simulink model "DHM"  (R2022a)
settings: Solver=FixedStepDiscrete  StartTime=0.0  StopTime=10.0  FixedStep=0.01  RelTol=1e-3
libraries: simulink x8, DoorHndDriver x4, DoorHndReq x4, DoorHndPosSts x4
(part 2 of 2)

== stateflow chart DHM/DHM_Step_sys/DHM/DoorHndSetSts ==
  state DrvDoorHndSet [parallel]
    settings: executionOrder=1
    (default) -> (junction 2)
    DrvDoorHndSet -> (junction 2)
    (junction 2) -> (junction 3) [order 1] : [hasChanged(SI_e_DrvDoorHndSet)]
    (junction 2) -> (junction 4) [order 2]
    (junction 3) -> (junction 39) : {SL_e_DrvDoorHndSetBackup = ...
        | SI_e_DrvDoorHndSet;}
    (junction 4) -> (junction 5) [order 1] : [SL_e_DrvDoorHndSetBackup == 4]
    (junction 4) -> (junction 43) [order 2]
    (junction 5) -> (junction 27)
    (junction 43) -> (junction 17) [order 1] : [SL_e_DrvDoorHndSetBackup == 3]
    (junction 27) -> (junction 6) [order 1] : [SI_m_FLDoorHndPosSts == Hnd_Unfold]
    (junction 43) -> (junction 26) [order 2]
    (junction 17) -> (junction 14) : {SO_b_DrvDoorHndBtnSetSts = 1;}
    (junction 27) -> (junction 8) [order 2]
    (junction 6) -> (junction 47) : {SO_b_DrvDoorHndSetSts = 1;}
    (junction 26) -> (junction 46) [order 1] : [SL_e_DrvDoorHndSetBackup == 6]
    (junction 26) -> (junction 42) [order 2]
    (junction 46) -> (junction 18) : {SO_b_DrvDoorHndBtnSetSts = 1;}
    (junction 14) -> (junction 28) [order 1] : [SI_m_FLDoorHndPosSts == Hnd_Unfold]
    (junction 14) -> (junction 20) [order 2]
    (junction 28) -> (junction 7) : {SO_b_DrvDoorHndSetSts = 1;}
    (junction 42) -> (junction 9) [order 1] : [SL_e_DrvDoorHndSetBackup == 5]
    (junction 42) -> (junction 19) [order 2] : {SO_b_DrvDoorHndSetSts = SI_b_DrvDoorHndSetFromEE;
        | SO_b_DrvDoorHndBtnSetSts = SI_b_DrvDoorHndBtnSetFromEE;}
    (junction 9) -> (junction 38) : {SO_b_DrvDoorHndSetSts = 0;
        | SO_b_DrvDoorHndBtnSetSts = 0;}
    (junction 12) -> (junction 19)
    (junction 38) -> (junction 12)
    (junction 18) -> (junction 38)
    (junction 20) -> (junction 18)
    (junction 7) -> (junction 20)
    (junction 8) -> (junction 7)
    (junction 47) -> (junction 8)
    (junction 39) -> (junction 47)
    (junction 19) -> (junction 29)
  state PassDoorHndSet [parallel]
    settings: executionOrder=2
    (default) -> (junction 79)
    PassDoorHndSet -> (junction 79)
    (junction 79) -> (junction 71) [order 1] : [hasChanged(SI_e_PassDoorHndSet)]
    (junction 79) -> (junction 83) [order 2]
    (junction 71) -> (junction 121) : {SL_e_PassDoorHndSetBackup = ...
        | SI_e_PassDoorHndSet;}
    (junction 83) -> (junction 73) [order 1] : [SL_e_PassDoorHndSetBackup == 4]
    (junction 83) -> (junction 77) [order 2]
    (junction 73) -> (junction 78)
    (junction 77) -> (junction 82) [order 1] : [SL_e_PassDoorHndSetBackup == 3]
    (junction 77) -> (junction 67) [order 2]
    (junction 82) -> (junction 72) : {SO_b_PassDoorHndBtnSetSts = 1;}
    (junction 78) -> (junction 74) [order 1] : [SI_m_FRDoorHndPosSts == Hnd_Unfold && ...
        | SI_m_RLDoorHndPosSts == Hnd_Unfold && ...
        | SI_m_RRDoorHndPosSts == Hnd_Unfold]
    (junction 78) -> (junction 106) [order 2]
    (junction 74) -> (junction 100) : {SO_b_PassDoorHndSetSts = 1;}
    (junction 67) -> (junction 75) [order 1] : [SL_e_PassDoorHndSetBackup == 6]
    (junction 67) -> (junction 68) [order 2]
    (junction 75) -> (junction 107) : {SO_b_PassDoorHndBtnSetSts = 1;}
    (junction 72) -> (junction 80) [order 1] : [SI_m_FRDoorHndPosSts == Hnd_Unfold && ...
        | SI_m_RLDoorHndPosSts == Hnd_Unfold && ...
        | SI_m_RRDoorHndPosSts == Hnd_Unfold]
    (junction 72) -> (junction 89) [order 2]
    (junction 80) -> (junction 110) : {SO_b_PassDoorHndSetSts = 1;}
    (junction 68) -> (junction 81) [order 1] : [SL_e_PassDoorHndSetBackup == 5]
    (junction 68) -> (junction 69) [order 2] : {SO_b_PassDoorHndSetSts = SI_b_PassDoorHndSetFromEE;
        | SO_b_PassDoorHndBtnSetSts = SI_b_PassDoorHndBtnSetFromEE;}
    (junction 81) -> (junction 88) : {SO_b_PassDoorHndSetSts = 0;
        | SO_b_PassDoorHndBtnSetSts = 0;}
    (junction 70) -> (junction 69)
    (junction 88) -> (junction 70)
    (junction 107) -> (junction 88)
    (junction 89) -> (junction 107)
    (junction 110) -> (junction 89)
    (junction 106) -> (junction 110)
    (junction 100) -> (junction 106)
    (junction 121) -> (junction 100)
    (junction 69) -> (junction 104)
  data: SI_e_DrvDoorHndSet input uint8; SI_e_PassDoorHndSet input uint8; SL_e_DrvDoorHndSetBackup local uint8 =0; SI_m_FLDoorHndPosSts input Enum: HndPos_Sts_E; SI_m_FRDoorHndPosSts input Enum: HndPos_Sts_E; SI_m_RLDoorHndPosSts input Enum: HndPos_Sts_E; SI_m_RRDoorHndPosSts input Enum: HndPos_Sts_E; SI_b_DrvDoorHndSetFromEE input boolean; SI_b_DrvDoorHndBtnSetFromEE input boolean; SO_b_DrvDoorHndSetSts output boolean; SO_b_DrvDoorHndBtnSetSts output boolean; SI_b_PassDoorHndSetFromEE input boolean; SI_b_PassDoorHndBtnSetFromEE input boolean; SO_b_PassDoorHndSetSts output boolean; SO_b_PassDoorHndBtnSetSts output boolean; SL_e_PassDoorHndSetBackup local uint8 =0

== stateflow chart DHM/DHM_Step_sys/DHM/HndPosSts ==
  state HndPosSts
    (default) -> (junction 70)
    HndPosSts -> (junction 70)
    (junction 70) -> (junction 71) : {SI_m_FLDoorHndPosSts = GetHndPosSts(SI_b_FLDoorHndPos1, SI_b_FLDoorHndPos2);}
    (junction 71) -> (junction 73)
    (junction 73) -> (junction 72) : {SI_m_FRDoorHndPosSts = GetHndPosSts(SI_b_FRDoorHndPos1, SI_b_FRDoorHndPos2);}
    (junction 72) -> (junction 74)
    (junction 74) -> (junction 75) : {SI_m_RLDoorHndPosSts = GetHndPosSts(SI_b_RLDoorHndPos1, SI_b_RLDoorHndPos2);}
    (junction 75) -> (junction 79)
    (junction 79) -> (junction 76) : {SI_m_RRDoorHndPosSts = GetHndPosSts(SI_b_RRDoorHndPos1, SI_b_RRDoorHndPos2);}
    (junction 76) -> (junction 80)
  state status = GetHndPosSts(pos1, pos2) [function]
    (default) -> (junction 37)
    (junction 37) -> (junction 38) [order 1] : [pos1 == 0 && pos2 == 0]
    (junction 37) -> (junction 39) [order 2]
    (junction 38) -> (junction 46) : {status = Hnd_Fold;}
    (junction 39) -> (junction 40) [order 1] : [pos1 == 1 && pos2 == 1]
    (junction 39) -> (junction 41) [order 2]
    (junction 40) -> (junction 45) : {status = Hnd_Unfold;}
    (junction 41) -> (junction 42) [order 1] : [pos1 == 1 && pos2 == 0]
    (junction 41) -> (junction 43) [order 2] : {status = Hnd_Error;}
    (junction 42) -> (junction 44) : {status = Hnd_Half_Unfold;}
    (junction 44) -> (junction 43)
    (junction 45) -> (junction 44)
    (junction 46) -> (junction 45)
    (junction 43) -> (junction 47)
  data: pos1 function_input double; pos2 function_input double; status function_output double; SI_b_FLDoorHndPos1 input boolean; SI_b_FLDoorHndPos2 input boolean; SI_b_FRDoorHndPos1 input boolean; SI_b_FRDoorHndPos2 input boolean; SI_b_RLDoorHndPos1 input boolean; SI_b_RLDoorHndPos2 input boolean; SI_b_RRDoorHndPos1 input boolean; SI_b_RRDoorHndPos2 input boolean; SI_m_FLDoorHndPosSts output Enum: HndPos_Sts_E; SI_m_FRDoorHndPosSts output Enum: HndPos_Sts_E; SI_m_RLDoorHndPosSts output Enum: HndPos_Sts_E; SI_m_RRDoorHndPosSts output Enum: HndPos_Sts_E
